simulink library "DaVinci_Lib"  (R2023a)
settings: Solver=VariableStepAuto  StartTime=0.0  StopTime=10.0  RelTol=1e-3
settings Model: Creator=ASUS  LastModifiedBy=ASUS

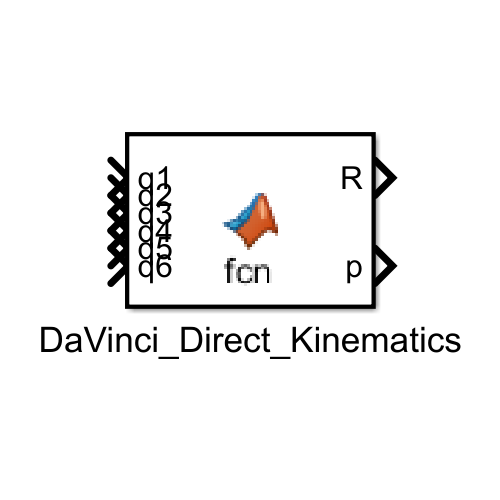
[thumbnail: Simulink's stored preview of the top-level diagram]
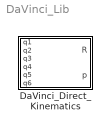
== system DaVinci_Lib ==
  DaVinci_Direct_Kinematics : MATLAB Function  TreatAsAtomicUnit=on

== matlab function DaVinci_Lib/DaVinci_Direct_Kinematics ==
  data: q1 input; R output; q2 input; q3 input; q4 input; q5 input; q6 input; p output
function [R,p] = DaVinci_Direct_Kinematics(q1,q2,q3,q4,q5,q6)
%#codegen

%    This function was generated by the Symbolic Math Toolbox version 9.3.
%    16-May-2023 12:09:14

% q1 = complex(q1);  % if required to enforce complex operations
% q2 = complex(q2);  % if required to enforce complex operations
% q3 = complex(q3);  % if required to enforce complex operations
% q4 = complex(q4);  % if required to enforce complex operations
% q5 = complex(q5);  % if required to enforce complex operations
% q6 = complex(q6);  % if required to enforce complex operations
t2 = cos(q1);
t3 = cos(q2);
t4 = cos(q4);
t5 = cos(q5);
t6 = cos(q6);
t7 = sin(q1);
t8 = sin(q2);
t9 = sin(q4);
t10 = sin(q5);
t11 = sin(q6);
R = reshape([-t7.*t9.*t11-t2.*t3.*t5.*t6+t2.*t4.*t8.*t11-t4.*t6.*t7.*t10-t2.*t6.*t8.*t9.*t10,t2.*t9.*t11-t3.*t5.*t6.*t7+t2.*t4.*t6.*t10+t4.*t7.*t8.*t11-t6.*t7.*t8.*t9.*t10,t3.*t4.*t11+t5.*t6.*t8-t3.*t6.*t9.*t10,-t6.*t7.*t9+t2.*t4.*t6.*t8+t2.*t3.*t5.*t11+t4.*t7.*t10.*t11+t2.*t8.*t9.*t10.*t11,t2.*t6.*t9+t4.*t6.*t7.*t8+t3.*t5.*t7.*t11-t2.*t4.*t10.*t11+t7.*t8.*t9.*t10.*t11,t3.*t4.*t6-t5.*t8.*t11+t3.*t9.*t10.*t11,t2.*t3.*t10-t4.*t5.*t7-t2.*t5.*t8.*t9,t2.*t4.*t5+t3.*t7.*t10-t5.*t7.*t8.*t9,-t8.*t10-t3.*t5.*t9],[3,3]);
if nargout > 1
    mt1 = [-q3.*t2.*t3-(t2.*t3.*t5)./1.0e+2-(t4.*t7.*t10)./1.0e+2-(t7.*t9.*t11)./5.0e+1-(t2.*t3.*t5.*t6)./5.0e+1+(t2.*t4.*t8.*t11)./5.0e+1-(t4.*t6.*t7.*t10)./5.0e+1-(t2.*t8.*t9.*t10)./1.0e+2-(t2.*t6.*t8.*t9.*t10)./5.0e+1;-q3.*t3.*t7-(t3.*t5.*t7)./1.0e+2+(t2.*t4.*t10)./1.0e+2+(t2.*t9.*t11)./5.0e+1-(t3.*t5.*t6.*t7)./5.0e+1+(t2.*t4.*t6.*t10)./5.0e+1+(t4.*t7.*t8.*t11)./5.0e+1-(t7.*t8.*t9.*t10)./1.0e+2-(t6.*t7.*t8.*t9.*t10)./5.0e+1];
    mt2 = [q3.*t8+(t5.*t8)./1.0e+2+(t3.*t4.*t11)./5.0e+1+(t5.*t6.*t8)./5.0e+1-(t3.*t9.*t10)./1.0e+2-(t3.*t6.*t9.*t10)./5.0e+1];
    p = [mt1;mt2];
end
end
